simulink model "demo6"  (Simulink 7.1)
settings: Solver=ode45  StartTime=0.0  StopTime=20.0  RelTol=1e-3
undefined symbols (not defined in the file): cond, gcamera, visjac
libraries: roblocks x4, simulink x1
settings Model: Creator=pic  LastModifiedBy=pic  ExtModeTrigMode=oneshot  ExtModeArmWhenConnect=off
settings DataIOCC: LimitDataPoints=off
settings OptimizationCC: BlockReduction=off  BooleanDataType=off
settings DebuggingCC: SaveWithParameterizedLinksMsg=none  SignalResolutionControl=TryResolveAllWithWarning  SolverPrmCheckMsg=none  MultiTaskDSMMsg=warning  MultiTaskCondExecSysMsg=none  StrictBusMsg=None
settings HardwareCC: TargetUnknown=on
settings RTWCC: IncludeERTFirstTime=on
settings GRTTargetCC: ModelReferenceCompliant=off  CompOptLevelCompliant=off  MatFileLogging=off

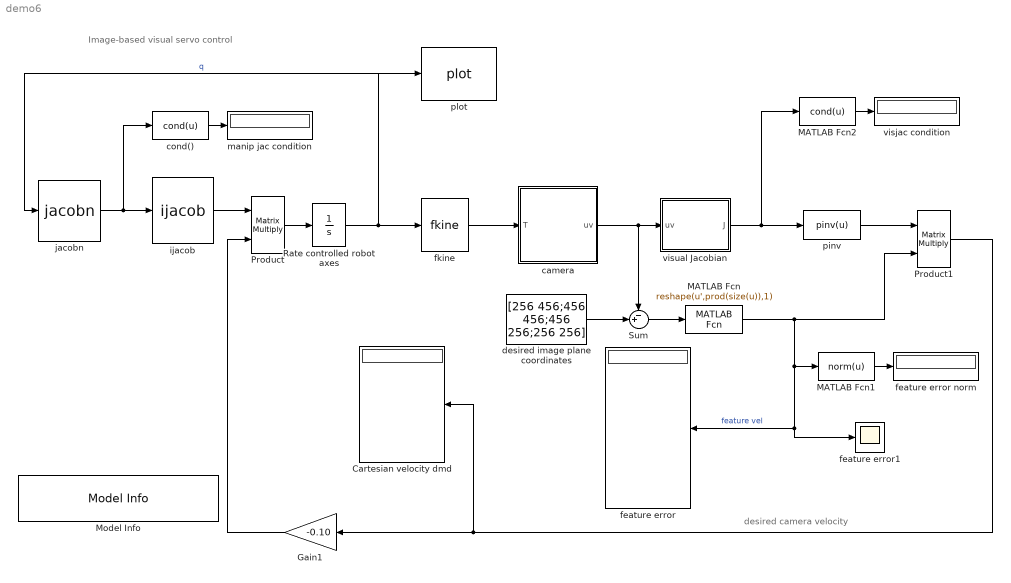
== system demo6 ==
  note: Image-based visual servo control
  note: desired camera velocity
  Cartesian velocity dmd : Display
      settings: Format=bank
  Gain1 : Gain  Orientation=left  Gain=-0.10  SaturateOnIntegerOverflow=on  OutDataTypeStr=Inherit: Same as input  ParamDataTypeStr=Inherit: Same as input
  MATLAB Fcn : MATLABFcn  MATLABFcn=reshape(u',prod(size(u)),1)
  MATLAB Fcn1 : MATLABFcn  MATLABFcn=norm(u)
  MATLAB Fcn2 : MATLABFcn  MATLABFcn=cond(u)
  Model Info : simulink/Model-Wide Utilities/Model Info  SystemSampleTime=-1  InitialBlockCM=none  BlockCM=none  Frame=on  DisplayStringWithTags=|  HorizontalTextAlignment=Left  LeftAlignmentValue=0.02  SourceBlockDiagram=demo6  TagMaxNumber=20
      | Image-based visual servo control
      | %<Creator>
      | %<LastModificationDate>
  Product : Product  Multiplication=Matrix(*)  SaturateOnIntegerOverflow=on  RndMeth=Zero  InputSameDT=on  OutDataTypeStr=Inherit: Same as first input
  Product1 : Product  Multiplication=Matrix(*)  SaturateOnIntegerOverflow=on  RndMeth=Zero  InputSameDT=on  OutDataTypeStr=Inherit: Same as first input
  Rate controlled robot axes : Integrator  InitialCondition="[0.3048   -0.9869    0.4483   -0.3513   -1.0595    0.1774]"
  Sum : Sum  Inputs=-+|  SaturateOnIntegerOverflow=on  InputSameDT=on  OutDataTypeStr=Inherit: Same as first input
  camera : Subsystem  mask{cam_name=IBVS camera, camdata=[8e-3 80e3 80e3 256 256], dims=[0 511 0 511], points=rotz(0.02)*[2 0.2 0.2;2 0.2 -0.2; 2 -0.2 -0.2 ;2 -0.2 0.2]}
      mask prompts: cam_name "Name"; camdata "Camera params"; dims "Image plane size"; points "Points (nx2)"
      mask init:
      | h=gcamera(cam_name,camcalp_c(camdata),dims);
  cond() : MATLABFcn  MATLABFcn=cond(u)
  desired image plane coordinates : Constant  Value=[256 456;456 456;456 256;256 256]  VectorParams1D=off
  feature error : Display
      settings: Format=bank
  feature error norm : Display
  feature error1 : Scope
      settings: YMin=10  YMax=55
  fkine : roblocks/fkine  SystemSampleTime=-1  robot=p560
  ijacob : roblocks/ijacob  SystemSampleTime=-1
  jacobn : roblocks/jacobn  SystemSampleTime=-1  robot=p560
  manip jac condition : Display
  pinv : MATLABFcn  MATLABFcn=pinv(u)  Output1D=off
  plot : roblocks/plot  SystemSampleTime=-1  robot=p560
  visjac condition : Display
  visual Jacobian : Subsystem  mask{camdata=[8e-3 80e3 80e3 256 256], z=2}
      mask prompts: camdata "Camera params"; z "Assumed depth (m)"
  wires:
  Rate controlled robot axes/1 -> fkine/1, plot/1, jacobn/1  "q"
  jacobn/1 -> ijacob/1, cond()/1
  Product/1 -> Rate controlled robot axes/1
  camera/1(uv) -> visual Jacobian/1(uv), Sum/1
  fkine/1 -> camera/1(T)
  visual Jacobian/1(J) -> pinv/1, MATLAB Fcn2/1
  Sum/1 -> MATLAB Fcn/1
  pinv/1 -> Product1/1
  desired image plane coordinates/1 -> Sum/2
  MATLAB Fcn/1 -> Product1/2, MATLAB Fcn1/1, feature error/1, feature error1/1  "feature vel"
  ijacob/1 -> Product/1
  MATLAB Fcn2/1 -> visjac condition/1
  cond()/1 -> manip jac condition/1
  MATLAB Fcn1/1 -> feature error norm/1
  Product1/1 -> Gain1/1, Cartesian velocity dmd/1
  Gain1/1 -> Product/2

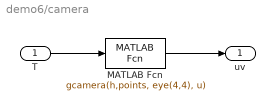
== system demo6/camera ==
  T : Inport
  MATLAB Fcn : MATLABFcn  MATLABFcn=gcamera(h,points, eye(4,4), u)  OutputDimensions=[4,2]  OutputSignalType=real  Output1D=off
  uv : Outport
  wires:
  MATLAB Fcn/1 -> uv/1
  T/1 -> MATLAB Fcn/1

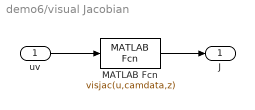
== system demo6/visual Jacobian ==
  uv : Inport
  MATLAB Fcn : MATLABFcn  MATLABFcn=visjac(u,camdata,z)  OutputDimensions=[8 6]  Output1D=off
  J : Outport
  wires:
  MATLAB Fcn/1 -> J/1
  uv/1 -> MATLAB Fcn/1
